simulink model "tut07"  (R2024b)
settings: Solver=VariableStepAuto  StartTime=0.0  StopTime=10.0  RelTol=1e-3
libraries: NSA_DEVS_SINKS x4, NSA_DEVS_LOGISTICS x2, NSA_DEVS_SOURCES x1, tutLib x1, NSA_DEVS_DIGITAL_LOGIC x1
settings Model: Creator=peter  LastModifiedBy=peter

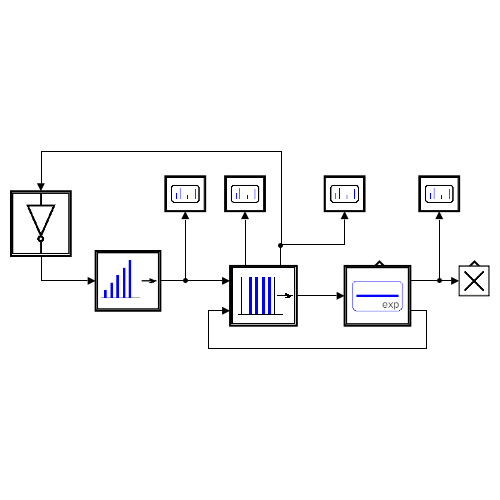
[thumbnail: Simulink's stored preview of the top-level diagram]
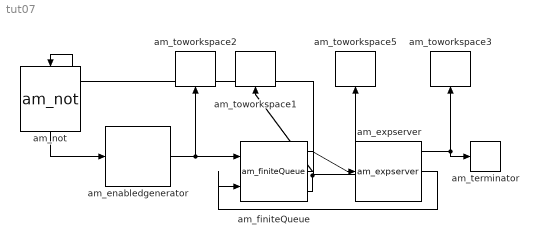
== system tut07 ==
  am_enabledgenerator : NSA_DEVS_SOURCES/am_enabledgenerator  tG=1  n0=1  nG=inf  tD=[0,2]  tau=[0,1]  debug=0
      settings: SourceProductName=Sources
  am_expserver : NSA_DEVS_LOGISTICS/am_expserver  tS=1  useSeed=false  seed=0  tau=[0,1]  debug=0
      settings: SourceProductName=Logistics
  am_finiteQueue : tutLib/am_finiteQueue  capacity=8  tD=[0,2]  tau=[0,1]  debug=0
  am_not : NSA_DEVS_DIGITAL_LOGIC/am_not  tau=[0,1]  debug=0
      settings: SourceProductName=Logic
  am_terminator : NSA_DEVS_LOGISTICS/am_terminator  tau=[0,1]  debug=0
      settings: SourceProductName=Logistics
  am_toworkspace1 : NSA_DEVS_SINKS/am_toworkspace  varname="\"qLen\""  t0=0  format="\"vector\""  tau=[0,5]  debug=0
      settings: SourceProductName=Sinks
  am_toworkspace2 : NSA_DEVS_SINKS/am_toworkspace  varname="\"gen\""  t0=0  format="\"vector\""  tau=[0,0.5]  debug=0
      settings: SourceProductName=Sinks
  am_toworkspace3 : NSA_DEVS_SINKS/am_toworkspace  varname="\"srvOut\""  t0=0  format="\"vector\""  tau=[0,5]  debug=0
      settings: SourceProductName=Sinks
  am_toworkspace5 : NSA_DEVS_SINKS/am_toworkspace  varname="\"isFull\""  t0=0  format="\"vector\""  tau=[0,5]  debug=0
      settings: SourceProductName=Sinks
  wires:
  am_enabledgenerator/1 -> am_finiteQueue/1, am_toworkspace2/1
  am_finiteQueue/1 -> am_expserver/1
  am_expserver/2 -> am_finiteQueue/2
  am_expserver/1 -> am_toworkspace3/1, am_terminator/1
  am_finiteQueue/2 -> am_toworkspace1/1
  am_finiteQueue/3 -> am_not/1, am_toworkspace5/1
  am_not/1 -> am_enabledgenerator/1
